simulink model "RV_Propogation"  (Simulink 6.4)
settings: Solver=ode45  StartTime=0.0  StopTime=8072.28  RelTol=1e-12
undefined symbols (not defined in the file or in its folder): Rint, Vint
settings Model: LastModifiedBy=C09Shankar.Kulumani

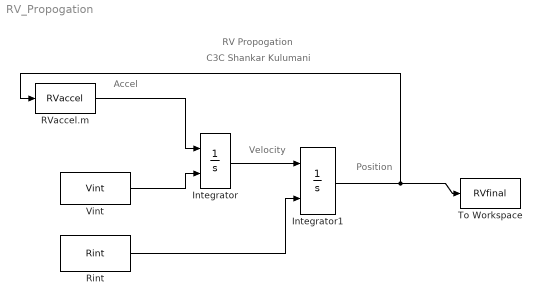
== system RV_Propogation ==
  note: Accel
  note: Velocity
  note: Position
  note: RV Propogation
  note: C3C Shankar Kulumani
  Integrator : Integrator  InitialConditionSource=external
  Integrator1 : Integrator  InitialConditionSource=external
  RVaccel.m : MATLABFcn  MATLABFcn=RVaccel
  Rint : Constant  Value=Rint  OutDataType=sfix(16)  ConRadixGroup=Use specified scaling  OutScaling=2^0  SampleTime=inf  FramePeriod=inf
  To Workspace : ToWorkspace  VariableName=RVfinal  SampleTime=-1  SaveFormat=Array
  Vint : Constant  Value=Vint  OutDataType=sfix(16)  ConRadixGroup=Use specified scaling  OutScaling=2^0  SampleTime=inf  FramePeriod=inf
  wires:
  RVaccel.m/1 -> Integrator/1
  Vint/1 -> Integrator/2
  Rint/1 -> Integrator1/2
  Integrator/1 -> Integrator1/1
  Integrator1/1 -> RVaccel.m/1, To Workspace/1
